simulink model "model_T_PSH_IEEE39"  (R2020b)
settings: Solver=ode3  StartTime=0.0  StopTime=300  FixedStep=Ts  RelTol=1e-3
PostLoadFcn:
  | IEEE39BusLineLength;
  | vNomHV = 345E3;fNom=60;load('Dynamicload.mat');
InitFcn:
  | IEEE39BusLineLength;
  | vNomHV = 345E3;fNom=60;load('Dynamicload.mat');
values from neighbouring files (symbols this model uses):
  At = 1.48    [MAIN_T_PSH_IEEE39.m]
  Dturb = 0.3    [MAIN_T_PSH_IEEE39.m]
  fix_mode = 1    [MAIN_T_PSH_IEEE39.m]
  Gmax = 1    [MAIN_T_PSH_IEEE39.m]
  Gmin = 0    [MAIN_T_PSH_IEEE39.m]
  Hdam = 1    [MAIN_T_PSH_IEEE39.m]
  Kd = 1    [MAIN_T_PSH_IEEE39.m]    (also in plots_T_PSH_IEEE39.m)
  max_delay_gen2pump = 20    [MAIN_T_PSH_IEEE39.m]
  max_delay_pump2hsc = 30    [MAIN_T_PSH_IEEE39.m]
  pgen_pump = Kd*Pref    (= 0.9)    [MAIN_T_PSH_IEEE39.m]
  pgen_turb = (1-Kd)*Pref    (= 0)    [MAIN_T_PSH_IEEE39.m]
  pgen_turb_gen2pump = (1-kd_gen2pump)*Pref    (= 0)    [MAIN_T_PSH_IEEE39.m]
  pgen_turb_hsc2gen = (1-kd_hsc2gen)*Pref    (= 0.36)    [MAIN_T_PSH_IEEE39.m]
  pgen_turb_pump2hsc = (1-kd_pump2hsc)*Pref    (= 0.36)    [MAIN_T_PSH_IEEE39.m]
  Pref = 0.9    [MAIN_T_PSH_IEEE39.m]    (also in MAIN_VS_PSH.m = 1)
  qNL = 0.1    [MAIN_T_PSH_IEEE39.m]
  R = 0.04    [MAIN_T_PSH_IEEE39.m]
  r = 0.31    [MAIN_T_PSH_IEEE39.m]
  Rp = 0.05    [IEEE39BusLineLength.m]
  Sn = 320E6    (= 320000000)    [MAIN_T_PSH_IEEE39.m]
  t_gen2pump = 10    [MAIN_T_PSH_IEEE39.m]
  t_hsc2gen = 150    [MAIN_T_PSH_IEEE39.m]
  t_pump2hsc = 35    [MAIN_T_PSH_IEEE39.m]
  t_sw_off = 220    [MAIN_FS_PSH_IEEE39.m]    (also in MAIN_T_PSH_IEEE39.m; MAIN_VS_PSH.m = 45)
  t_sw_on = 130    [MAIN_FS_PSH_IEEE39.m]    (also in MAIN_T_PSH_IEEE39.m; MAIN_VS_PSH.m = 35)
  Tf = 0.05    [MAIN_T_PSH_IEEE39.m]
  Tg = 0.5    [MAIN_T_PSH_IEEE39.m]
  TL_10_11_len = 14    [IEEE39BusLineLength.m]
  TL_10_13_len = 14    [IEEE39BusLineLength.m]
  TL_13_14_len = 32    [IEEE39BusLineLength.m]
  TL_14_15_len = 70    [IEEE39BusLineLength.m]
  TL_15_16_len = 31.5    [IEEE39BusLineLength.m]
  TL_16_17_len = 26    [IEEE39BusLineLength.m]
  TL_16_19_len = 61    [IEEE39BusLineLength.m]
  TL_16_21_len = 46    [IEEE39BusLineLength.m]
  TL_16_24_len = 15    [IEEE39BusLineLength.m]
  TL_17_18_len = 26    [IEEE39BusLineLength.m]
  TL_17_27_len = 59    [IEEE39BusLineLength.m]
  TL_1_2_len = 134    [IEEE39BusLineLength.m]
  TL_1_39_len = 105    [IEEE39BusLineLength.m]
  TL_21_22_len = 47    [IEEE39BusLineLength.m]
  TL_22_23_len = 33    [IEEE39BusLineLength.m]
  TL_24_23_len = 88    [IEEE39BusLineLength.m]
  TL_25_26_len = 101    [IEEE39BusLineLength.m]
  TL_26_27_len = 46.5    [IEEE39BusLineLength.m]
  TL_26_28_len = 151    [IEEE39BusLineLength.m]
  TL_26_29_len = 200    [IEEE39BusLineLength.m]
  TL_28_29_len = 48    [IEEE39BusLineLength.m]
  TL_2_25_len = 28    [IEEE39BusLineLength.m]
  TL_2_2_len = 49    [IEEE39BusLineLength.m]
  TL_3_18_len = 42    [IEEE39BusLineLength.m]
  TL_3_4_len = 53    [IEEE39BusLineLength.m]
  TL_4_14_len = 33    [IEEE39BusLineLength.m]
  TL_4_5_len = 32.5    [IEEE39BusLineLength.m]
  TL_5_6_len = 14    [IEEE39BusLineLength.m]
  TL_5_8_len = 32    [IEEE39BusLineLength.m]
  TL_6_11_len = 26.5    [IEEE39BusLineLength.m]
  TL_6_7_len = 25.5    [IEEE39BusLineLength.m]
  TL_7_8_len = 15    [IEEE39BusLineLength.m]
  TL_8_9_len = 93    [IEEE39BusLineLength.m]
  TL_9_39_len = 136    [IEEE39BusLineLength.m]
  Tr = 6.88    [MAIN_T_PSH_IEEE39.m]
  Ts = 25e-6    (= 2.5e-05)    [MAIN_FS_PSH_IEEE39.m]    (also in MAIN_T_PSH_IEEE39.m; MAIN_VS_PSH.m = 1e-07)
  Velm = 0.05    [MAIN_T_PSH_IEEE39.m]
  Vn = 18000    [MAIN_T_PSH_IEEE39.m]
undefined symbols (not defined in the file or in its folder): D1, Delta, load15, load16, load18, load20, load21, load23, load24, load25, load26, load27, load28, load29, load3, load39, load4, load7, load8
libraries: powerlib x216, sps_avr x10, simulink_extras x7, powerlib_meascontrol x5, simulink x1
(part 2 of 9)

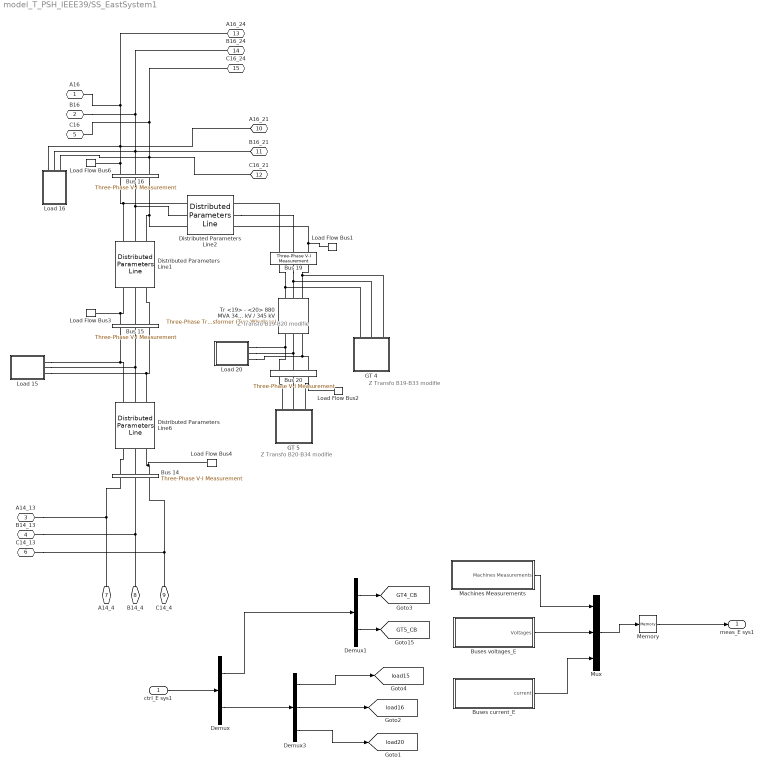
== system model_T_PSH_IEEE39/SS_EastSystem1 ==
  note: Z Transfo B19-B20 modifie
  note: Z Transfo B20-B34 modifie
  note: Z Transfo B19-B33 modifie
  ctrl_E sys1 : Inport
  Bus 14 : powerlib/Measurements/Three-Phase V-I Measurement  VoltageMeasurement=phase-to-ground  SetLabelV=on  LabelV=V_bus_14  Vpu=off  VpuLL=off  CurrentMeasurement=yes  SetLabelI=on  LabelI=I_bus_14  Ipu=off  Pbase=100e6  Vbase=230e3  OutputType=Complex  PhasorSimulation=off  PSBequivalent=0
  Bus 15 : powerlib/Measurements/Three-Phase V-I Measurement  VoltageMeasurement=phase-to-ground  SetLabelV=on  LabelV=V_bus_15  Vpu=off  VpuLL=off  CurrentMeasurement=yes  SetLabelI=on  LabelI=I_bus_15  Ipu=off  Pbase=100e6  Vbase=230e3  OutputType=Complex  PhasorSimulation=off  PSBequivalent=0
  Bus 16 : powerlib/Measurements/Three-Phase V-I Measurement  VoltageMeasurement=phase-to-ground  SetLabelV=on  LabelV=V_bus_16  Vpu=off  VpuLL=off  CurrentMeasurement=yes  SetLabelI=on  LabelI=I_bus_16  Ipu=off  Pbase=100e6  Vbase=230e3  OutputType=Complex  PhasorSimulation=off  PSBequivalent=0
  Bus 19 : powerlib/Measurements/Three-Phase V-I Measurement  VoltageMeasurement=phase-to-ground  SetLabelV=on  LabelV=V_bus_19  Vpu=off  VpuLL=off  CurrentMeasurement=yes  SetLabelI=on  LabelI=I_bus_19  Ipu=off  Pbase=100e6  Vbase=230e3  OutputType=Complex  PhasorSimulation=off  PSBequivalent=0
  Bus 20 : powerlib/Measurements/Three-Phase V-I Measurement  VoltageMeasurement=phase-to-ground  SetLabelV=on  LabelV=V_bus_20  Vpu=off  VpuLL=off  CurrentMeasurement=yes  SetLabelI=on  LabelI=I_bus_20  Ipu=off  Pbase=100e6  Vbase=230e3  OutputType=Complex  PhasorSimulation=off  PSBequivalent=0
  Buses current_E : Subsystem
  Buses voltages_E : Subsystem
  Demux : Demux  Outputs=[2 6]
  Demux1 : Demux  Outputs=2
  Demux3 : Demux  Outputs=[2 2 2]
  Distributed Parameters Line1 : powerlib/Elements/Distributed Parameters Line  Phases=3  Length=TL_15_16_len  Frequency=fNom  Resistance=[1.071 4.285]/TL_15_16_len  Inductance=[0.03 0.089]/TL_15_16_len  Capacitance=[0.381e-6 0.173e-6]/TL_15_16_len  x1=[-0.000125 3.55201829698564e-08 245444.290173048 -3207.76452881805;-0.0001 3.52355613436191e-08 245403.151295772 -5520.83756553109;-7.5e-05 3.49478098910877e-08 245340.214291653 -7833.42020952954;-5e-05 3.465695417201e-08 245255.484751118 -10145.3070438513;-2.5e-05 3.43630200218728e-08 245148.970200335 -12456.2927133403]  x2=[-0.000125 2.34646584577738e-08 242476.39429401 2987.47863299293;-0.0001 2.32370672989382e-08 242493.775143427 702.101999990364;-7.5e-05 2.30074120894261e-08 242489.616293613 -1583.33699777147;-5e-05 2.27757132285409e-08 242463.918113979 -3868.63535438615;-2.5e-05 2.25419912971154e-08 242416.682887189 -6153.59007643981]  x3=[-0.000125 -1.71237451775812e-10 305.815637466811 -202.156893770744;-0.0001 -1.74723912247073e-10 303.896797052738 -205.030084840958;-7.5e-05 -1.78194852730176e-10 301.950962767989 -207.885063953531;-5e-05 -1.8164996491612e-10 299.978307452816 -210.721577512712;-2.5e-05 -1.85088941901861e-10 297.979006329871 -213.539373562965]  x4=[-0.000125 2.55868113259471e-10 1428.03590450797 236.352811737226;-0.0001 2.58654787659917e-10 1430.19998246802 222.883619968435;-7.5e-05 2.61418486846554e-10 1432.23702179607 209.394630387783;-5e-05 2.64158965331642e-10 1434.14684155051 195.88704116532;-2.5e-05 2.66875979690036e-10 1435.9292720901 182.362052123222]  x5=0.000124084648526721  V1=ones(3,3)  V2=ones(3,3)  I1=ones(3,3)  I2=ones(3,3)  nHarmo=1  Measurements=None  Decoupling=off  VsMag0=0  VrMag0=0  VsAngle0=0  VrAngle0=0  IsMag0=0  IrMag0=0  IsAngle0=0  IrAngle0=0
  Distributed Parameters Line2 : powerlib/Elements/Distributed Parameters Line  Phases=3  Length=TL_16_19_len  Frequency=fNom  Resistance=[1.904 7.618]/TL_16_19_len  Inductance=[0.062 0.185]/TL_16_19_len  Capacitance=[0.677e-6 0.308e-6]/TL_16_19_len  x1=[-0.00025 3.68954687011655e-08 115423.439527174 -216634.791494799;-0.000225 3.66268697942173e-08 117460.007707478 -215537.345336034;-0.0002 3.63550174769137e-08 119486.142410732 -214420.753903997;-0.000175 3.60799358967494e-08 121501.663663936 -213285.116380796;-0.00015 3.5801649488061e-08 123506.392436839 -212130.533640322;-0.000125 3.55201829698564e-08 125500.150657839 -210957.10823929;-0.0001 3.52355613436191e-08 127482.761229804 -209764.944408129;-7.5e-05 3.49478098910877e-08 129454.048045797 -208554.148041724;-5e-05 3.465695417201e-08 131413.836004727 -207324.826690009;-2.5e-05 3.43630200218728e-08 133361.951026895 -206077.089548415]  x2=[-0.00025 1.39707369421026e-07 130491.434683277 -207401.001286105;-0.000225 1.39176513308374e-07 132440.310284365 -206161.954000369;-0.0002 1.38633294733077e-07 134377.421771311 -204904.594217829;-0.000175 1.38077761946951e-07 136302.59707867 -203629.033624452;-0.00015 1.37509964295629e-07 138215.665201243 -202335.385522905;-0.000125 1.36929952214181e-07 140116.456209255 -201023.764822493;-0.0001 1.36337777222636e-07 142004.801263459 -199694.288028949;-7.5e-05 1.35733491921398e-07 143880.532630129 -198347.07323409;-5e-05 1.35117149986584e-07 145743.483695959 -196982.240105324;-2.5e-05 1.34488806165247e-07 147593.488982863 -195599.90987502]  x3=[-0.00025 5.93365044472736e-10 795.636520838787 -1334.36307084348;-0.000225 6.06302735018928e-10 808.177011788381 -1326.80514289647;-0.0002 6.19186570250493e-10 820.645715782827 -1319.12936044495;-0.000175 6.3201540575069e-10 833.041525279741 -1311.3364052963;-0.00015 6.4478810198817e-10 845.36333921165 -1303.42696966585;-0.000125 6.57503524418203e-10 857.610063083794 -1295.40175611541;-0.0001 6.70160543583446e-10 869.780609071348 -1287.26147749084;-7.5e-05 6.82758035214272e-10 881.873896116046 -1279.00685685877;-5e-05 6.95294880328635e-10 893.888850022207 -1270.63862744233;-2.5e-05 7.07769965331462e-10 905.824403552154 -1262.15753255604]  x4=[-0.00025 -3.61483614737921e-10 -40.8192622512322 -91.5404410367902;-0.000225 -3.75361793747798e-10 -39.9547127392966 -91.921156465683;-0.0002 -3.89206630952775e-10 -39.0866142187533 -92.2937069259612;-0.000175 -4.03016896574359e-10 -38.2150437991324 -92.6580593255388;-0.00015 -4.16791363904905e-10 -37.3400788983581 -93.0141813005289;-0.000125 -4.30528809416579e-10 -36.4617972358719 -93.3620412181185;-0.0001 -4.44228012870041e-10 -35.5802768257294 -93.7016081793784;-7.5e-05 -4.57887757422828e-10 -34.6955959696706 -94.0328520220078;-5e-05 -4.71506829737447e-10 -33.8078332501643 -94.3557433230131;-2.5e-05 -4.8508402008915e-10 -32.9170675234284 -94.6702534013221]  x5=0.000238704838660635  V1=ones(3,3)  V2=ones(3,3)  I1=ones(3,3)  I2=ones(3,3)  nHarmo=1  Measurements=None  Decoupling=off  VsMag0=0  VrMag0=0  VsAngle0=0  VrAngle0=0  IsMag0=0  IrMag0=0  IsAngle0=0  IrAngle0=0
  Distributed Parameters Line6 : powerlib/Elements/Distributed Parameters Line  Phases=3  Length=TL_14_15_len  Frequency=fNom  Resistance=[2.142 8.57]/TL_14_15_len  Inductance=[0.069 0.206]/TL_14_15_len  Capacitance=[0.816e-6 0.371e-6]/TL_14_15_len  x1=[-0.0003 2.50001359282586e-08 0 0;-0.000275 2.47875505343122e-08 0 0;-0.00025 2.45727633668034e-08 242066.515546201 14406.3225173659;-0.000225 2.43557935043701e-08 242191.533476518 12124.3019718169;-0.0002 2.41366602195301e-08 242295.038554456 9841.20447566275;-0.000175 2.39153829769688e-08 242377.021586096 7557.23282682426;-0.00015 2.36919814318103e-08 242437.47528923 5272.58990086941;-0.000125 2.34664754278717e-08 242476.39429401 2987.47863299293;-0.0001 2.32388849959e-08 242493.775143427 702.101999990361;-7.5e-05 2.30092303517934e-08 242489.616293613 -1583.33699777147;-5e-05 2.27775318948054e-08 242463.918113979 -3868.63535438615;-2.5e-05 2.25438102057324e-08 242416.682887189 -6153.59007643981]  x2=[-0.0003 1.03135232680497e-09 0 0;-0.000275 8.59599046141902e-10 0 0;-0.00025 6.8776941092127e-10 241274.041685216 2466.16253916518;-0.000225 5.15878684044808e-10 241286.563136279 192.141492105228;-0.0002 3.43942133840767e-10 241277.65211966 -2081.89662207303;-0.000175 1.71975032707689e-10 241247.309426888 -4355.74981015559;-0.00015 -7.34424216934234e-15 241195.537753177 -6629.21609535462;-0.000125 -1.7198972053967e-10 241122.341697186 -8902.09353524927;-0.0001 -3.43956819715731e-10 241027.727760612 -11174.1802397233;-7.5e-05 -5.15893366658272e-10 240911.704347612 -13445.2743888982;-5e-05 -6.87784088969038e-10 240774.281764055 -15715.17425106;-2.5e-05 -8.59613718320187e-10 240615.472216612 -17983.6782005781]  x3=[-0.0003 -5.32719529297102e-11 0 0;-0.000275 -5.63436805761488e-11 0 0;-0.00025 -5.94104034510938e-11 1278.02817822225 18.8054041271025;-0.000225 -6.24718491504874e-11 1278.14864980591 6.75964667004504;-0.0002 -6.55277457390209e-11 1278.1555888361 -5.28671121791455;-0.000175 -6.85778217742899e-11 1278.04899469647 -17.3325995096155;-0.00015 -7.16218063309051e-11 1277.82887685532 -29.3769482196092;-0.000125 -7.46594290245575e-11 1277.4952548648 -41.4186874992015;-0.0001 -7.76904200360355e-11 1277.04815835914 -53.4567477314832;-7.5e-05 -8.07145101351922e-11 1276.48762705202 -65.4900596263391;-5e-05 -8.37314307048593e-11 1275.8137107331 -77.5175543154288;-2.5e-05 -8.67409137647076e-11 1275.0264692635 -89.53816344713]  x4=[-0.0003 8.89875620705852e-11 0 0;-0.000275 9.15590501678496e-11 0 0;-0.00025 9.41224054608744e-11 372.387444854488 113.017323741447;-0.000225 9.6677400257621e-11 373.436019719486 109.502718488205;-0.0002 9.92238076086783e-11 374.451423837968 105.97838657035;-0.000175 1.01761401327422e-10 375.43356701587 102.444641039423;-0.00015 1.04289956010105e-10 376.382362013554 98.9017957831332;-0.000125 1.0680924705588e-10 377.297724553564 95.350165497482;-0.0001 1.0931905068675e-10 378.179573328105 91.7900656588071;-7.5e-05 1.11819143967444e-10 379.027830006271 88.2218124957609;-5e-05 1.14309304825221e-10 379.842419240999 84.6457229612216;-2.5e-05 1.16789312069596e-10 380.623268675763 81.0621147041387]  x5=0.000276452527570286  V1=ones(3,3)  V2=ones(3,3)  I1=ones(3,3)  I2=ones(3,3)  nHarmo=1  Measurements=None  Decoupling=off  VsMag0=0  VrMag0=0  VsAngle0=0  VrAngle0=0  IsMag0=0  IrMag0=0  IsAngle0=0  IrAngle0=0
  GT 4 : Subsystem
  GT 5 : Subsystem
  Load 15 : Subsystem
  Load 16 : Subsystem
  Load 20 : Subsystem
  Load Flow Bus1 : powerlib/Measurements/Load Flow Bus  LConnTagsString=a  Phases=single  Connectors=on one side  ID=Bus-19  Vbase=345e+003  Vref=1  Vangle=0  VLF=1.019  VLFb=1  VLFc=1  angleLF=21.55  angleLFb=0  angleLFc=0
      settings: AttributesFormatString=%<ID>\n%<Vbase>V\n%<VLF>pu\n%<angleLF>deg.
  Load Flow Bus2 : powerlib/Measurements/Load Flow Bus  LConnTagsString=a  Phases=single  Connectors=on one side  ID=Bus-20  Vbase=345e+003  Vref=1  Vangle=0  VLF=0.9613  VLFb=1  VLFc=1  angleLF=-10.55  angleLFb=0  angleLFc=0
      settings: AttributesFormatString=%<ID>\n%<Vbase>V\n%<VLF>pu\n%<angleLF>deg.
  Load Flow Bus3 : powerlib/Measurements/Load Flow Bus  LConnTagsString=a  Phases=single  Connectors=on one side  ID=Bus-15  Vbase=345e+003  Vref=1  Vangle=0  VLF=0.996  VLFb=1  VLFc=1  angleLF=18.53  angleLFb=0  angleLFc=0
      settings: AttributesFormatString=%<ID>\n%<Vbase>V\n%<VLF>pu\n%<angleLF>deg.
  Load Flow Bus4 : powerlib/Measurements/Load Flow Bus  LConnTagsString=a  Phases=single  Connectors=on one side  ID=Bus-14  Vbase=345e+003  Vref=1  Vangle=0  VLF=1.001  VLFb=1  VLFc=1  angleLF=20.12  angleLFb=0  angleLFc=0
      settings: AttributesFormatString=%<ID>\n%<Vbase>V\n%<VLF>pu\n%<angleLF>deg.
  Load Flow Bus6 : powerlib/Measurements/Load Flow Bus  LConnTagsString=a  Phases=single  Connectors=on one side  ID=Bus-16  Vbase=345e+003  Vref=1  Vangle=0  VLF=1.007  VLFb=1  VLFc=1  angleLF=19.22  angleLFb=0  angleLFc=0
      settings: AttributesFormatString=%<ID>\n%<Vbase>V\n%<VLF>pu\n%<angleLF>deg.
  Machines Measurements : Subsystem
      mask Display: disp('Machines Measurements')
  Memory : Memory
  Mux : Mux  Inputs=3
  Tr <19> - <20> 880 MVA 345 kV / 345 kV : powerlib/Elements/Three-Phase Transformer (Two Windings)  Winding1Connection=Delta (D1)  Winding2Connection=Yg  CoreType=Three single-phase transformers  SetSaturation=off  Hysteresis=off  DataFile='hysteresis'  SetInitialFlux=off  Measurements=None  UNITS=pu  NominalPower=[ 880e6 fNom]  Winding1="[ 345e3 0.0007*880/100/2   0.0138*880/100/2 ]"  Winding2="[ 1.06*345e3 0.0007*880/100/2   0.0138*880/100/2 ]"  Rm=500  Lm=500  L0=0.5  Saturation="[ 0,0  ;  0.005,1.2  ;  1.0,1.4 ]"  InitialFluxes=[ 0.8 , -0.8 , 0.7 ]  BreakLoop=off  DiscreteSolver=Trapezoidal iterative  DataType=off  TransfoNumber=0
  A16 : PMIOPort  Side=Left
  B16 : PMIOPort  Port=2  Side=Left
  A14_13 : PMIOPort  Port=3  Side=Right
  B14_13 : PMIOPort  Port=4  Side=Right
  C16 : PMIOPort  Port=5  Side=Left
  C14_13 : PMIOPort  Port=6  Side=Right
  A14_4 : PMIOPort  Port=7  Side=Right
  B14_4 : PMIOPort  Port=8  Side=Right
  C14_4 : PMIOPort  Port=9  Side=Right
  A16_21 : PMIOPort  Port=10  Side=Left
  B16_21 : PMIOPort  Port=11  Side=Left
  C16_21 : PMIOPort  Port=12  Side=Left
  A16_24 : PMIOPort  Port=13  Side=Left
  B16_24 : PMIOPort  Port=14  Side=Left
  C16_24 : PMIOPort  Port=15  Side=Left
  meas_E sys1 : Outport
  tag scope: GT4_CB=global, GT5_CB=global, load15=global, load16=global, load20=global
  wires:
  Machines Measurements/1(Machines Measurements) -> Mux/1
  Mux/1 -> Memory/1
  Memory/1 -> meas_E sys1/1
  Buses voltages_E/1(Voltages) -> Mux/2
  Buses current_E/1(current) -> Mux/3
  ctrl_E sys1/1 -> Demux/1
  Demux/1 -> Demux1/1
  Demux1/2 -> [GT5_CB]
  Demux/2 -> Demux3/1
  Demux3/1 -> [load15]
  Demux3/2 -> [load16]
  Demux3/3 -> [load20]
  Demux1/1 -> [GT4_CB]
  connections:
  A14_4/RConn1 -- A14_13/RConn1 -- Bus 14/LConn1
  C14_4/RConn1 -- Bus 14/LConn3 -- C14_13/RConn1
  B14_4/RConn1 -- B14_13/RConn1 -- Bus 14/LConn2
  Tr <19> - <20> 880 MVA 345 kV / 345 kV/LConn3 -- Load 20/LConn3 -- Bus 20/RConn3
  Load 20/LConn2 -- Tr <19> - <20> 880 MVA 345 kV / 345 kV/LConn2 -- Bus 20/RConn2
  Load 20/LConn1 -- Tr <19> - <20> 880 MVA 345 kV / 345 kV/LConn1 -- Bus 20/RConn1
  GT 5/RConn3 -- Bus 20/LConn3 -- Load Flow Bus2/LConn1
  Bus 20/LConn2 -- GT 5/RConn2
  GT 5/RConn1 -- Bus 20/LConn1
  GT 4/RConn3 -- Tr <19> - <20> 880 MVA 345 kV / 345 kV/RConn3 -- Bus 19/LConn3
  GT 4/RConn2 -- Tr <19> - <20> 880 MVA 345 kV / 345 kV/RConn2 -- Bus 19/LConn2
  GT 4/RConn1 -- Tr <19> - <20> 880 MVA 345 kV / 345 kV/RConn1 -- Bus 19/LConn1
  C16/RConn1 -- C16_24/RConn1 -- Load 16/LConn3 -- Bus 16/RConn3 -- C16_21/RConn1
  B16/RConn1 -- B16_24/RConn1 -- Load 16/LConn2 -- B16_21/RConn1 -- Bus 16/RConn2
  Load Flow Bus6/LConn1 -- Bus 16/RConn1 -- Load 16/LConn1 -- A16_21/RConn1 -- A16_24/RConn1 -- A16/RConn1
  Bus 15/RConn3 -- Distributed Parameters Line1/RConn1
  Bus 15/RConn2 -- Distributed Parameters Line1/RConn2
  Bus 15/RConn1 -- Distributed Parameters Line1/RConn3 -- Load Flow Bus3/LConn1
  Bus 14/RConn3 -- Distributed Parameters Line6/RConn1 -- Load Flow Bus4/LConn1
  Bus 14/RConn2 -- Distributed Parameters Line6/RConn2
  Bus 14/RConn1 -- Distributed Parameters Line6/RConn3
  Bus 16/LConn1 -- Distributed Parameters Line2/LConn1 -- Distributed Parameters Line1/LConn3
  Bus 16/LConn2 -- Distributed Parameters Line1/LConn2 -- Distributed Parameters Line2/LConn2
  Bus 16/LConn3 -- Distributed Parameters Line2/LConn3 -- Distributed Parameters Line1/LConn1
  Load 15/LConn1 -- Distributed Parameters Line6/LConn3 -- Bus 15/LConn1
  Load 15/LConn2 -- Distributed Parameters Line6/LConn2 -- Bus 15/LConn2
  Bus 15/LConn3 -- Load 15/LConn3 -- Distributed Parameters Line6/LConn1
  Bus 19/RConn1 -- Distributed Parameters Line2/RConn1
  Distributed Parameters Line2/RConn2 -- Bus 19/RConn2
  Bus 19/RConn3 -- Distributed Parameters Line2/RConn3 -- Load Flow Bus1/LConn1

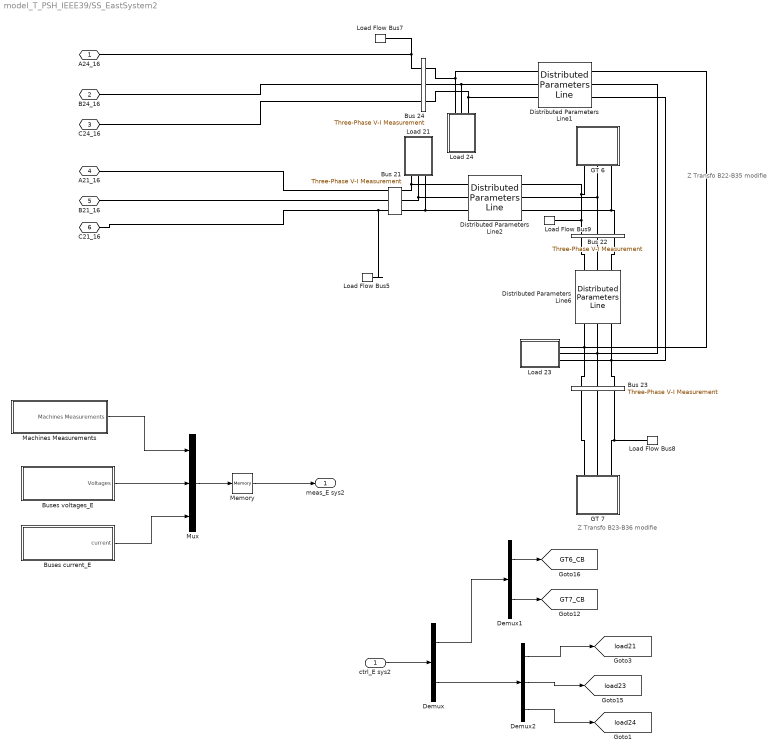
== system model_T_PSH_IEEE39/SS_EastSystem2 ==
  note: Z Transfo B22-B35 modifie
  note: Z Transfo B23-B36 modifie
  ctrl_E sys2 : Inport
  Bus 21 : powerlib/Measurements/Three-Phase V-I Measurement  VoltageMeasurement=phase-to-ground  SetLabelV=on  LabelV=V_bus_21  Vpu=off  VpuLL=off  CurrentMeasurement=yes  SetLabelI=on  LabelI=I_bus_21  Ipu=off  Pbase=100e6  Vbase=230e3  OutputType=Complex  PhasorSimulation=off  PSBequivalent=0
  Bus 22 : powerlib/Measurements/Three-Phase V-I Measurement  VoltageMeasurement=phase-to-ground  SetLabelV=on  LabelV=V_bus_22  Vpu=off  VpuLL=off  CurrentMeasurement=yes  SetLabelI=on  LabelI=I_bus_22  Ipu=off  Pbase=100e6  Vbase=230e3  OutputType=Complex  PhasorSimulation=off  PSBequivalent=0
  Bus 23 : powerlib/Measurements/Three-Phase V-I Measurement  VoltageMeasurement=phase-to-ground  SetLabelV=on  LabelV=V_bus_23  Vpu=off  VpuLL=off  CurrentMeasurement=yes  SetLabelI=on  LabelI=I_bus_23  Ipu=off  Pbase=100e6  Vbase=230e3  OutputType=Complex  PhasorSimulation=off  PSBequivalent=0
  Bus 24 : powerlib/Measurements/Three-Phase V-I Measurement  VoltageMeasurement=phase-to-ground  SetLabelV=on  LabelV=V_bus_24  Vpu=off  VpuLL=off  CurrentMeasurement=yes  SetLabelI=on  LabelI=I_bus_24  Ipu=off  Pbase=100e6  Vbase=230e3  OutputType=Complex  PhasorSimulation=off  PSBequivalent=0
  Buses current_E : Subsystem
  Buses voltages_E : Subsystem
  Demux : Demux  Outputs=[2 6]
  Demux1 : Demux  Outputs=2
  Demux2 : Demux  Outputs=[2 2 2]
  Distributed Parameters Line1 : powerlib/Elements/Distributed Parameters Line  Phases=3  Length=TL_24_23_len  Frequency=fNom  Resistance=[2.619 10.474]/TL_24_23_len  Inductance=[0.111 0.332]/TL_24_23_len  Capacitance=[0.805e-6 0.365e-6]/TL_24_23_len  x1=[-0.00035 3.18356926291058e-08 107249.073525914 -222796.923832124;-0.000325 3.16302590802303e-08 109344.080602946 -221776.24491419;-0.0003 3.14220159488539e-08 111429.3751065 -220735.866547849;-0.000275 3.12109817323357e-08 113504.771808661 -219675.881145525;-0.00025 3.0997175175955e-08 115570.086360695 -218596.38286125;-0.000225 3.07806152712464e-08 117625.13530942 -217497.467582303;-0.0002 3.05613212543128e-08 119669.736113506 -216379.232920693;-0.000175 3.03393126041168e-08 121703.707159688 -215241.778204488;-0.00015 3.01146090407503e-08 123726.867778898 -214085.204468994;-0.000125 2.98872305236831e-08 125739.03826231 -212909.614447777;-0.0001 2.96571972499899e-08 127740.039877308 -211715.112563539;-7.5e-05 2.9424529652556e-08 129729.694883358 -210501.804918846;-5e-05 2.91892483982628e-08 131707.826547799 -209269.799286697;-2.5e-05 2.89513743861516e-08 133674.259161538 -208019.205100957]  x2=[-0.00035 3.88919473158324e-09 129221.537910763 -201084.863578238;-0.000325 3.97039374423041e-09 131110.940867007 -199858.066964586;-0.0003 4.051240083548e-09 132988.697791386 -198613.517801826;-0.000275 4.13172656829669e-09 134854.641890674 -197351.326638012;-0.00025 4.21184604920153e-09 136708.607420926 -196071.605588261;-0.000225 4.29159140958696e-09 138550.429702204 -194774.468324795;-0.0002 4.37095556600898e-09 140379.945133203 -193460.030066848;-0.000175 4.44993146888432e-09 142196.991205785 -192128.407570424;-0.00015 4.52851210311665e-09 144001.40651941 -190779.719117935;-0.000125 4.60669048871966e-09 145793.030795478 -189414.084507686;-0.0001 4.68445968143712e-09 147571.70489156 -188031.62504324;-7.5e-05 4.76181277335966e-09 149337.27081554 -186632.46352264;-5e-05 4.83874289353839e-09 151089.571739643 -185216.724227501;-2.5e-05 4.91524320859522e-09 152828.452014368 -183784.532911976]  x3=[-0.00035 -2.23651488499992e-10 802.285172053634 -1103.14082645126;-0.000325 -2.25732028830483e-10 812.646229468615 -1095.53058575592;-0.0003 -2.27792518336969e-10 822.935102946692 -1087.82303369948;-0.000275 -2.29832773994857e-10 833.150878570632 -1080.01885491128;-0.00025 -2.31852614576842e-10 843.292648916176 -1072.11874260362;-0.000225 -2.33851860669006e-10 853.35951313264 -1064.12339851013;-0.0002 -2.3583033468675e-10 863.350577022937 -1056.03353282353;-0.000175 -2.37787860890572e-10 873.264953123004 -1047.84986413244;-0.00015 -2.39724265401677e-10 883.101760780628 -1039.57311935766;-0.000125 -2.41639376217419e-10 892.860126233677 -1031.20403368749;-0.0001 -2.43533023226582e-10 902.539182687707 -1022.74335051252;-7.5e-05 -2.4540503822449e-10 912.138070392958 -1014.19182135956;-5e-05 -2.47255254927946e-10 921.655936720724 -1005.55020582487;-2.5e-05 -2.49083508990005e-10 931.091936239082 -996.819271506703]  x4=[-0.00035 2.61421164614829e-10 -232.992471385861 -68.1394715347156;-0.000325 2.63388449065466e-10 -232.339973510927 -70.3323182735123;-0.0003 2.6533233783112e-10 -231.666837856133 -72.5189176891314;-0.000275 2.67252658244348e-10 -230.973124213279 -74.6990755551696;-0.00025 2.6914923973119e-10 -230.258894202023 -76.8725982173995;-0.000225 2.71021913826311e-10 -229.524211264404 -79.0392926109707;-0.0002 2.7287051418797e-10 -228.769140659208 -81.198966277559;-0.000175 2.74694876612795e-10 -227.993749456173 -83.351427382462;-0.00015 2.76494839050365e-10 -227.198106530028 -85.4964847316385;-0.000125 2.78270241617609e-10 -226.382282554379 -87.633947788692;-0.0001 2.80020926613007e-10 -225.546349995429 -89.7636266917945;-7.5e-05 2.81746738530594e-10 -224.69038310554 -91.885332270552;-5e-05 2.83447524073776e-10 -223.814457916641 -93.998876062807;-2.5e-05 2.85123132168949e-10 -222.918652233473 -96.1040703313791]  x5=0.000348109178276012  V1=ones(3,3)  V2=ones(3,3)  I1=ones(3,3)  I2=ones(3,3)  nHarmo=1  Measurements=None  Decoupling=off  VsMag0=0  VrMag0=0  VsAngle0=0  VrAngle0=0  IsMag0=0  IrMag0=0  IsAngle0=0  IrAngle0=0
  Distributed Parameters Line2 : powerlib/Elements/Distributed Parameters Line  Phases=3  Length=TL_21_22_len  Frequency=fNom  Resistance=[0.9522 3.809]/TL_21_22_len  Inductance=[0.044 0.133]/TL_21_22_len  Capacitance=[0.572e-6 0.26e-6]/TL_21_22_len  x1=[-0.0002 1.49365973206953e-08 0 0;-0.000175 1.46837342890637e-08 127042.880582269 -205846.70751626;-0.00015 1.44295669632497e-08 128977.258914018 -204640.23140741;-0.000125 1.41741179198648e-08 130900.180739872 -203415.577969956;-0.0001 1.39174098493701e-08 132811.475254794 -202172.855984697;-7.5e-05 1.36594655540607e-08 134710.972686554 -200912.175837386;-5e-05 1.34003079460404e-08 136598.504310808 -199633.649508922;-2.5e-05 1.31399600451864e-08 138473.902466083 -198337.390565408]  x2=[-0.0002 -6.3068411379596e-09 0 0;-0.000175 -6.50470370620221e-09 145589.79328016 -192435.442415383;-0.00015 -6.70198848905078e-09 147396.951575036 -191054.764235348;-0.000125 -6.89867796253018e-09 149191.017220409 -189657.115466456;-0.0001 -7.09475465554411e-09 150971.830856994 -188242.620255952;-7.5e-05 -7.29020115142694e-09 152739.234302629 -186811.404247478;-5e-05 -7.48500008949083e-09 154493.070566319 -185363.594569918;-2.5e-05 -7.67913416656775e-09 156233.183862187 -183899.319826096]  x3=[-0.0002 -1.22674308931313e-10 0 0;-0.000175 -1.2688420489242e-10 1303.52884091451 -1820.98656408738;-0.00015 -1.31082830264792e-10 1320.63306549039 -1808.62039981537;-0.000125 -1.35269812102245e-10 1337.61998380136 -1796.09358342182;-0.0001 -1.39444778492844e-10 1354.48808697111 -1783.40722761099;-7.5e-05 -1.43607358591934e-10 1371.2358766772 -1770.56245925837;-5e-05 -1.47757182655081e-10 1387.86186528409 -1757.56041931055;-2.5e-05 -1.51893882070917e-10 1404.36457597535 -1744.4022626839]  x4=[-0.0002 1.37610559762618e-10 0 0;-0.000175 1.41211814709251e-10 -365.947467183574 359.299846497004;-0.00015 1.44800526406001e-10 -369.317536493119 355.834967008835;-0.000125 1.48376376082744e-10 -372.654800883641 352.338480201423;-0.0001 1.51939046111836e-10 -375.958963920022 348.810696652944;-7.5e-05 1.55488220036325e-10 -379.229732107395 345.251929721529;-5e-05 1.59023582598063e-10 -382.466814917217 341.662495517435;-2.5e-05 1.62544819765704e-10 -385.669924813078 338.042712874962]  x5=0.000185956984273245  V1=ones(3,3)  V2=ones(3,3)  I1=ones(3,3)  I2=ones(3,3)  nHarmo=1  Measurements=None  Decoupling=off  VsMag0=0  VrMag0=0  VsAngle0=0  VrAngle0=0  IsMag0=0  IrMag0=0  IsAngle0=0  IrAngle0=0
  Distributed Parameters Line6 : powerlib/Elements/Distributed Parameters Line  Phases=3  Length=TL_22_23_len  Frequency=fNom  Resistance=[0.714 2.857]/TL_22_23_len  Inductance=[0.03 0.091]/TL_22_23_len  Capacitance=[0.411e-6 0.187e-6]/TL_22_23_len  x1=[-0.00015 4.52892332957795e-09 0 0;-0.000125 4.60703323325838e-09 145793.030795478 -189414.084507686;-0.0001 4.6847339136087e-09 147571.70489156 -188031.62504324;-7.5e-05 4.76201846880521e-09 149337.27081554 -186632.46352264;-5e-05 4.83888003398685e-09 151089.571739643 -185216.724227501;-2.5e-05 4.91531178186499e-09 152828.452014368 -183784.532911976]  x2=[-0.00015 -6.70198848905078e-09 0 0;-0.000125 -6.89867796253018e-09 149191.017220409 -189657.115466456;-0.0001 -7.09475465554411e-09 150971.830856994 -188242.620255952;-7.5e-05 -7.29020115142694e-09 152739.234302629 -186811.404247478;-5e-05 -7.48500008949083e-09 154493.070566319 -185363.594569918;-2.5e-05 -7.67913416656775e-09 156233.183862187 -183899.319826096]  x3=[-0.00015 8.23518814062508e-10 0 0;-0.000125 8.19887766249129e-10 521.39068045771 -1011.28001100054;-0.0001 8.16183891263679e-10 530.898421086645 -1006.32117888493;-7.5e-05 8.1240751810575e-10 540.359004248111 -1001.27295950356;-5e-05 8.0855898221464e-10 549.77158959841 -996.135801268464;-2.5e-05 8.04638625439562e-10 559.135341057287 -990.910160491744]  x4=[-0.00015 -8.27071322865471e-10 0 0;-0.000125 -8.23610156058685e-10 538.954191475565 -411.843321172881;-0.0001 -8.20075831435641e-10 542.811706117143 -406.745578987236;-7.5e-05 -8.16468662935488e-10 546.621005084391 -401.611707307421;-5e-05 -8.1278897096779e-10 550.381750013351 -396.442162153604;-2.5e-05 -8.09037082384063e-10 554.093606852911 -391.237402714676]  x5=0.000130449223838243  V1=ones(3,3)  V2=ones(3,3)  I1=ones(3,3)  I2=ones(3,3)  nHarmo=1  Measurements=None  Decoupling=off  VsMag0=0  VrMag0=0  VsAngle0=0  VrAngle0=0  IsMag0=0  IrMag0=0  IsAngle0=0  IrAngle0=0
  GT 6 : Subsystem
  GT 7 : Subsystem
  Load 21 : Subsystem
  Load 23 : Subsystem
  Load 24 : Subsystem
  Load Flow Bus5 : powerlib/Measurements/Load Flow Bus  LConnTagsString=a  Phases=single  Connectors=on one side  ID=Bus-21  Vbase=345e+003  Vref=1  Vangle=0  VLF=1.006  VLFb=1  VLFc=1  angleLF=20.56  angleLFb=0  angleLFc=0
      settings: AttributesFormatString=%<ID>\n%<Vbase>V\n%<VLF>pu\n%<angleLF>deg.
  Load Flow Bus7 : powerlib/Measurements/Load Flow Bus  LConnTagsString=a  Phases=single  Connectors=on one side  ID=Bus-24  Vbase=345e+003  Vref=1  Vangle=0  VLF=1.011  VLFb=1  VLFc=1  angleLF=19.08  angleLFb=0  angleLFc=0
      settings: AttributesFormatString=%<ID>\n%<Vbase>V\n%<VLF>pu\n%<angleLF>deg.
  Load Flow Bus8 : powerlib/Measurements/Load Flow Bus  LConnTagsString=a  Phases=single  Connectors=on one side  ID=Bus-23  Vbase=345e+003  Vref=1  Vangle=0  VLF=1.012  VLFb=1  VLFc=1  angleLF=23.42  angleLFb=0  angleLFc=0
      settings: AttributesFormatString=%<ID>\n%<Vbase>V\n%<VLF>pu\n%<angleLF>deg.
  Load Flow Bus9 : powerlib/Measurements/Load Flow Bus  LConnTagsString=a  Phases=single  Connectors=on one side  ID=Bus-22  Vbase=345e+003  Vref=1  Vangle=0  VLF=1.019  VLFb=1  VLFc=1  angleLF=23.66  angleLFb=0  angleLFc=0
      settings: AttributesFormatString=%<ID>\n%<Vbase>V\n%<VLF>pu\n%<angleLF>deg.
  Machines Measurements : Subsystem
      mask Display: disp('Machines Measurements')
  Memory : Memory
  Mux : Mux  Inputs=3
  A24_16 : PMIOPort  Side=Left
  B24_16 : PMIOPort  Port=2  Side=Left
  C24_16 : PMIOPort  Port=3  Side=Left
  A21_16 : PMIOPort  Port=4  Side=Left
  B21_16 : PMIOPort  Port=5  Side=Left
  C21_16 : PMIOPort  Port=6  Side=Left
  meas_E sys2 : Outport
  tag scope: GT6_CB=global, GT7_CB=global, load21=global, load23=global, load24=global
  wires:
  Machines Measurements/1(Machines Measurements) -> Mux/1
  Mux/1 -> Memory/1
  Memory/1 -> meas_E sys2/1
  Buses voltages_E/1(Voltages) -> Mux/2
  Buses current_E/1(current) -> Mux/3
  Demux/1 -> Demux1/1
  Demux/2 -> Demux2/1
  Demux1/2 -> [GT7_CB]
  Demux1/1 -> [GT6_CB]
  Demux2/1 -> [load21]
  Demux2/2 -> [load23]
  Demux2/3 -> [load24]
  ctrl_E sys2/1 -> Demux/1
  connections:
  Bus 24/RConn3 -- C24_16/RConn1
  Bus 24/RConn2 -- B24_16/RConn1
  Bus 24/RConn1 -- Load Flow Bus7/LConn1 -- A24_16/RConn1
  Load 23/LConn3 -- Distributed Parameters Line6/LConn3 -- Distributed Parameters Line1/RConn3 -- Bus 23/RConn3
  Load 23/LConn2 -- Distributed Parameters Line6/LConn2 -- Distributed Parameters Line1/RConn2 -- Bus 23/RConn2
  Load 23/LConn1 -- Distributed Parameters Line6/LConn1 -- Bus 23/RConn1 -- Distributed Parameters Line1/RConn1
  Load Flow Bus8/LConn1 -- GT 7/RConn3 -- Bus 23/LConn3
  Bus 22/RConn3 -- GT 6/RConn3 -- Distributed Parameters Line2/RConn3
  GT 6/RConn2 -- Bus 22/RConn2 -- Distributed Parameters Line2/RConn2
  Load Flow Bus9/LConn1 -- Distributed Parameters Line2/RConn1 -- GT 6/RConn1 -- Bus 22/RConn1
  Distributed Parameters Line6/RConn3 -- Bus 22/LConn3
  Distributed Parameters Line6/RConn2 -- Bus 22/LConn2
  Distributed Parameters Line6/RConn1 -- Bus 22/LConn1
  Bus 21/RConn1 -- Load 21/LConn1 -- Distributed Parameters Line2/LConn1
  Bus 21/RConn2 -- Load 21/LConn2 -- Distributed Parameters Line2/LConn2
  Bus 21/RConn3 -- Distributed Parameters Line2/LConn3 -- Load 21/LConn3
  C21_16/RConn1 -- Load Flow Bus5/LConn1 -- Bus 21/LConn3
  Load 24/LConn1 -- Distributed Parameters Line1/LConn1 -- Bus 24/LConn1
  Load 24/LConn2 -- Distributed Parameters Line1/LConn2 -- Bus 24/LConn2
  Bus 24/LConn3 -- Load 24/LConn3 -- Distributed Parameters Line1/LConn3
  Bus 21/LConn2 -- B21_16/RConn1
  A21_16/RConn1 -- Bus 21/LConn1
  GT 7/RConn1 -- Bus 23/LConn1
  GT 7/RConn2 -- Bus 23/LConn2
